simulink model "tst2"  (R2013b)
settings: Solver=VariableStepDiscrete  StartTime=0.0  StopTime=128  RelTol=1e-3
settings Model: Creator=eric  LastModifiedBy=eric

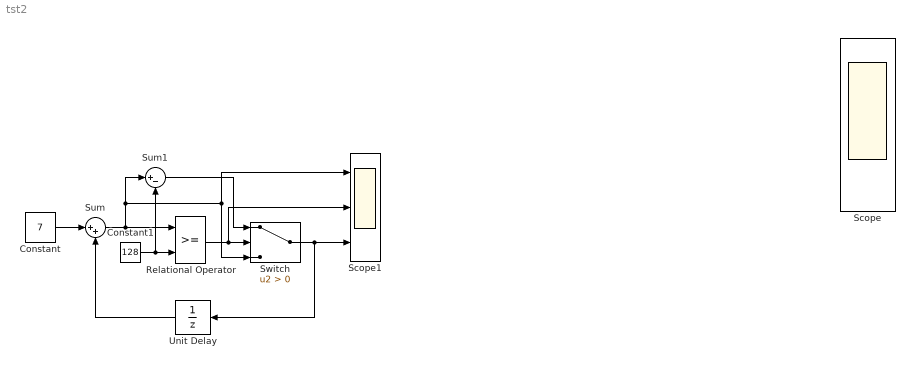
== system tst2 ==
  Constant : Constant  Value=7  SampleTime=1
  Constant1 : Constant  Value=128  SampleTime=1
  Relational Operator : RelationalOperator  OutDataTypeStr=boolean  SampleTime=1
  Scope : Scope  NumInputPorts=4
      settings: TimeRange=0.02  YMin=0.89999997~0.8~-0.2~-1  YMax=0.90000003~2~0.8~1  MaxDataPoints=20000
  Scope1 : Scope  NumInputPorts=3
      settings: YMin=-5~-5~-5  YMax=5~5~5
  Sum : Sum  Inputs=|++  SampleTime=1
  Sum1 : Sum  Inputs=|+-  SampleTime=1
  Switch : Switch  Criteria=u2 > Threshold  SampleTime=1
  Unit Delay : UnitDelay
  wires:
  Constant/1 -> Sum/1
  Constant1/1 -> Sum1/2, Relational Operator/2
  Relational Operator/1 -> Scope1/2, Switch/2
  Sum1/1 -> Switch/1
  Sum/1 -> Sum1/1, Scope1/1, Switch/3, Relational Operator/1
  Switch/1 -> Scope1/3, Unit Delay/1
  Unit Delay/1 -> Sum/2
